simulink model "Test_RC_Filters"  (R2017b)
settings: Solver=VariableStepAuto  StartTime=0.0  StopTime=1  MaxStep=1e-4  RelTol=1e-3
libraries: powerlib x48, powerlib_extras x2
settings Model: Creator=chemi  LastModifiedBy=chemi

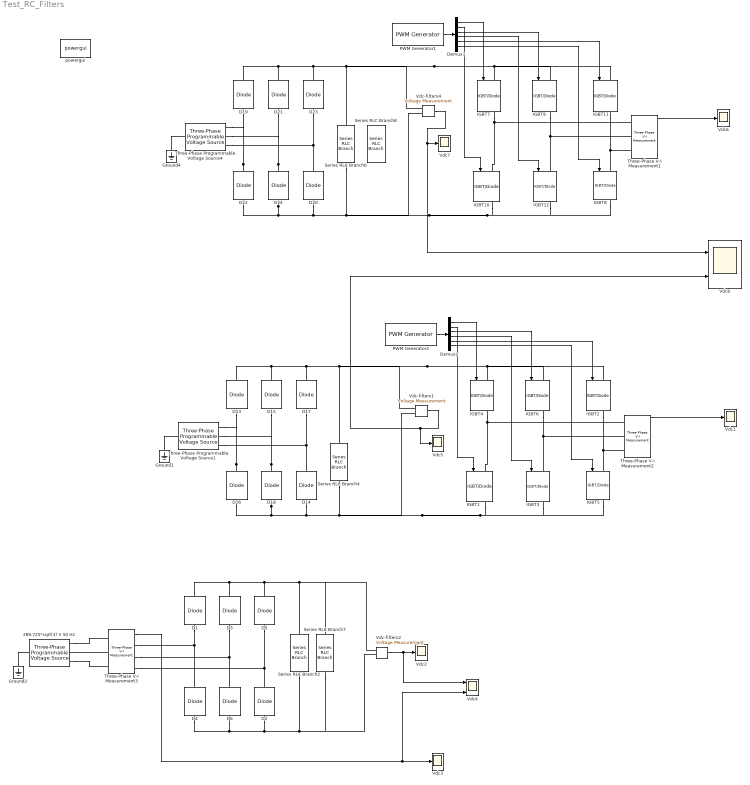
== system Test_RC_Filters ==
  289.725*sqrt(3) V 50 Hz : powerlib/Electrical Sources/Three-Phase Programmable Voltage Source  PositiveSequence=[289.725*sqrt(3) 0 50]  VariationEntity=None  VariationType=Table of time-amplitude pairs  VariationTypeAlt=Step  VariationStep=0.5  VariationRate=10  VariationMagnitude=0.3  VariationFrequency=2  VariationTiming=[1 2]  VariationPhaseA=off  Amplitudes=[1 0.8 1.2 1.0]  TimeValues=[0 0.1 0.15 0.2]  HarmonicGeneration=off  HarmonicA=[3 0.2 -25 0]  HarmonicB=[2 0.15 35 2]  Timing="[0.05  3]"  BusType=swing  Pref=0  Qref=0  Qmin=-inf  Qmax=inf
  D{1..6,13..24} (18 alike) : powerlib/Power Electronics/Diode  Ron=0.001  Lon=0  Vf=0  IC=0  UseSnubber=off  Rs=500  Cs=250e-9  Measurements=off
  Demux1 : Demux  Outputs=6
  Demux2 : Demux  Outputs=6
  Ground1 : powerlib/Elements/Ground  LConnTagsString=a
  Ground2 : powerlib/Elements/Ground  LConnTagsString=a
  Ground4 : powerlib/Elements/Ground  LConnTagsString=a
  IGBT{1..12} (12 alike) : powerlib/Power Electronics/IGBT//Diode  Ron=1e-3  Rs=1e5  Cs=inf  Measurements=on
  PWM Generator1 : powerlib_extras/Control  Blocks/PWM Generator  GeneratorMode="3-arm  bridge (6 pulses)"  Fc=5000  Internal=on  mIndex=1  Freq=50  Phase=0
  PWM Generator2 : powerlib_extras/Control  Blocks/PWM Generator  GeneratorMode="3-arm  bridge (6 pulses)"  Fc=5000  Internal=on  mIndex=1  Freq=50  Phase=0
  Series RLC Branch2 : powerlib/Elements/Series RLC Branch  LConnTagsString=__new0  RConnTagsString=__new0  BranchType=C  Resistance=3000  Inductance=200e-6  SetiL0=off  InitialCurrent=0  Capacitance=22000e-6  Setx0=off  InitialVoltage=0  Measurements=None
  Series RLC Branch4 : powerlib/Elements/Series RLC Branch  LConnTagsString=__new0  RConnTagsString=__new0  BranchType=C  Resistance=3000  Inductance=1e-3  SetiL0=off  InitialCurrent=0  Capacitance=3500e-6  Setx0=off  InitialVoltage=0  Measurements=None
  Series RLC Branch6 : powerlib/Elements/Series RLC Branch  LConnTagsString=__new0  RConnTagsString=__new0  BranchType=C  Resistance=3000  Inductance=1e-3  SetiL0=off  InitialCurrent=0  Capacitance=17000e-6  Setx0=off  InitialVoltage=0  Measurements=None
  Series RLC Branch7 : powerlib/Elements/Series RLC Branch  LConnTagsString=__new0  RConnTagsString=__new0  BranchType=R  Resistance=2200  Inductance=200e-6  SetiL0=off  InitialCurrent=0  Capacitance=10000e-6  Setx0=off  InitialVoltage=0  Measurements=None
  Series RLC Branch8 : powerlib/Elements/Series RLC Branch  LConnTagsString=__new0  RConnTagsString=__new0  BranchType=R  Resistance=3000  Inductance=200e-6  SetiL0=off  InitialCurrent=0  Capacitance=10000e-6  Setx0=off  InitialVoltage=0  Measurements=None
  Three-Phase Programmable Voltage Source1 : powerlib/Electrical Sources/Three-Phase Programmable Voltage Source  PositiveSequence=[289.725*sqrt(3) 0 50]  VariationEntity=None  VariationType=Table of time-amplitude pairs  VariationTypeAlt=Step  VariationStep=0.5  VariationRate=10  VariationMagnitude=0.3  VariationFrequency=2  VariationTiming=[1 2]  VariationPhaseA=off  Amplitudes=[1 0.8 1.2 1.0]  TimeValues=[0 0.1 0.15 0.2]  HarmonicGeneration=off  HarmonicA=[3 0.2 -25 0]  HarmonicB=[2 0.15 35 2]  Timing="[0.05  3]"  BusType=swing  Pref=0  Qref=0  Qmin=-inf  Qmax=inf
  Three-Phase Programmable Voltage Source4 : powerlib/Electrical Sources/Three-Phase Programmable Voltage Source  PositiveSequence=[289.725*sqrt(3) 0 50]  VariationEntity=None  VariationType=Table of time-amplitude pairs  VariationTypeAlt=Step  VariationStep=0.5  VariationRate=10  VariationMagnitude=0.3  VariationFrequency=2  VariationTiming=[1 2]  VariationPhaseA=off  Amplitudes=[1 0.8 1.2 1.0]  TimeValues=[0 0.1 0.15 0.2]  HarmonicGeneration=off  HarmonicA=[3 0.2 -25 0]  HarmonicB=[2 0.15 35 2]  Timing="[0.05  3]"  BusType=swing  Pref=0  Qref=0  Qmin=-inf  Qmax=inf
  Three-Phase V-I Measurement1 : powerlib/Measurements/Three-Phase V-I Measurement  VoltageMeasurement=phase-to-phase  SetLabelV=off  LabelV=Vabc  Vpu=off  VpuLL=off  CurrentMeasurement=yes  SetLabelI=off  LabelI=Iabc  Ipu=off  Pbase=100e6  Vbase=500e3  OutputType=Complex  PhasorSimulation=off  PSBequivalent=0
  Three-Phase V-I Measurement2 : powerlib/Measurements/Three-Phase V-I Measurement  VoltageMeasurement=phase-to-phase  SetLabelV=off  LabelV=Vabc  Vpu=off  VpuLL=off  CurrentMeasurement=yes  SetLabelI=off  LabelI=Iabc  Ipu=off  Pbase=100e6  Vbase=500e3  OutputType=Complex  PhasorSimulation=off  PSBequivalent=0
  Three-Phase V-I Measurement3 : powerlib/Measurements/Three-Phase V-I Measurement  VoltageMeasurement=phase-to-phase  SetLabelV=off  LabelV=Vabc  Vpu=off  VpuLL=off  CurrentMeasurement=no  SetLabelI=off  LabelI=Iabc  Ipu=off  Pbase=100e6  Vbase=500e3  OutputType=Complex  PhasorSimulation=off  PSBequivalent=0
  Vdc-filters1 : powerlib/Measurements/Voltage Measurement  PhasorSimulation=off  OutputType=Complex  PSBequivalent=0
  Vdc-filters2 : powerlib/Measurements/Voltage Measurement  PhasorSimulation=off  OutputType=Complex  PSBequivalent=0
  Vdc-filters4 : powerlib/Measurements/Voltage Measurement  PhasorSimulation=off  OutputType=Complex  PSBequivalent=0
  Vdc{1..3,5..7} (6 alike) : Scope
  Vdc4 : Scope  NumInputPorts=2
  Vdc8 : Scope  NumInputPorts=2
  powergui : powerlib/powergui  Priority=1  SimulationMode=Continuous  SampleTime=50e-6  frequency=60  Iterations=50  frequencyindice=50  Pbase=100e6  ErrMax=1e-4  UnitsV=kV  UnitsW=MW  buscounter=0  FunctionMessages=off  echomessages=off  EnableUseOfTLC=off  CurrentSourceSwitches=off  DisableSnubberDevices=off  DisableRonSwitches=off  DisableVfSwitches=off  DisplayEquations=off  SolverType=Tustin/Backward Euler (TBE)  Interpol=off  ExternalGateDelay=off  methode=off  Ts=100  x0status=blocks  SPID=on  SwTol=0  HookPort=off  RestoreLinks=warning  ResistiveCurrentMeasurement=off  Frange=[0:2:500]  Ylog=off  Xlog=on  ShowGrid=off  save=off  variable=ZData  structure=0  ZoomFFT=on  StartTime=0.0  cycles=1  DisplayStyle=1  fundamental=60  FreqAxis=off  MaxFrequency=1000  frequencyindicesteady=1  RmsSteady=1  display=off
  wires:
  Vdc-filters4/1 -> Vdc7/1, Vdc8/1
  Three-Phase V-I Measurement1/1 -> Vdc6/1
  Demux1/5 -> IGBT11/1
  Demux1/2 -> IGBT10/1
  Demux1/4 -> IGBT12/1
  Demux1/1 -> IGBT7/1
  Demux1/3 -> IGBT9/1
  PWM Generator1/1 -> Demux1/1
  Demux1/6 -> IGBT8/1
  Demux2/6 -> IGBT5/1
  PWM Generator2/1 -> Demux2/1
  Demux2/3 -> IGBT6/1
  Demux2/1 -> IGBT4/1
  Demux2/4 -> IGBT3/1
  Demux2/2 -> IGBT1/1
  Demux2/5 -> IGBT2/1
  Three-Phase V-I Measurement2/1 -> Vdc1/1
  Vdc-filters1/1 -> Vdc8/2, Vdc5/1
  Vdc-filters2/1 -> Vdc4/1, Vdc2/1
  Three-Phase V-I Measurement3/1 -> Vdc4/2, Vdc3/1
  connections:
  D23/RConn1 -- Vdc-filters4/LConn1 -- IGBT7/LConn1 -- IGBT11/LConn1 -- IGBT9/LConn1 -- Series RLC Branch6/LConn1 -- D21/RConn1 -- D19/RConn1
  D24/LConn1 -- D20/LConn1 -- IGBT8/RConn1 -- IGBT12/RConn1 -- IGBT10/RConn1 -- Vdc-filters4/LConn2 -- Series RLC Branch6/RConn1 -- D22/LConn1
  Three-Phase V-I Measurement1/LConn1 -- IGBT10/LConn1 -- IGBT7/RConn1
  Three-Phase V-I Measurement1/LConn2 -- IGBT12/LConn1 -- IGBT9/RConn1
  Three-Phase V-I Measurement1/LConn3 -- IGBT8/LConn1 -- IGBT11/RConn1
  D23/LConn1 -- D20/RConn1 -- Three-Phase Programmable Voltage Source4/RConn3
  D24/RConn1 -- D21/LConn1 -- Three-Phase Programmable Voltage Source4/RConn2
  D22/RConn1 -- D19/LConn1 -- Three-Phase Programmable Voltage Source4/RConn1
  Ground4/LConn1 -- Three-Phase Programmable Voltage Source4/LConn1
  D17/RConn1 -- D13/RConn1 -- D15/RConn1 -- IGBT6/LConn1 -- IGBT2/LConn1 -- IGBT4/LConn1 -- Vdc-filters1/LConn1 -- Series RLC Branch4/LConn1
  D18/LConn1 -- D16/LConn1 -- Vdc-filters1/LConn2 -- IGBT1/RConn1 -- IGBT3/RConn1 -- IGBT5/RConn1 -- Series RLC Branch4/RConn1 -- D14/LConn1
  Three-Phase V-I Measurement2/LConn1 -- IGBT4/RConn1 -- IGBT1/LConn1
  Three-Phase V-I Measurement2/LConn2 -- IGBT6/RConn1 -- IGBT3/LConn1
  Three-Phase V-I Measurement2/LConn3 -- IGBT2/RConn1 -- IGBT5/LConn1
  D17/LConn1 -- Three-Phase Programmable Voltage Source1/RConn3 -- D14/RConn1
  D18/RConn1 -- Three-Phase Programmable Voltage Source1/RConn2 -- D15/LConn1
  D16/RConn1 -- Three-Phase Programmable Voltage Source1/RConn1 -- D13/LConn1
  Ground1/LConn1 -- Three-Phase Programmable Voltage Source1/LConn1
  D5/RConn1 -- Series RLC Branch2/LConn1 -- Series RLC Branch7/LConn1 -- Vdc-filters2/LConn1 -- D1/RConn1 -- D3/RConn1
  D3/LConn1 -- Three-Phase V-I Measurement3/RConn2 -- D6/RConn1
  Series RLC Branch2/RConn1 -- Vdc-filters2/LConn2 -- Series RLC Branch7/RConn1 -- D2/LConn1 -- D4/LConn1 -- D6/LConn1
  D1/LConn1 -- Three-Phase V-I Measurement3/RConn1 -- D4/RConn1
  D5/LConn1 -- Three-Phase V-I Measurement3/RConn3 -- D2/RConn1
  Ground2/LConn1 -- 289.725*sqrt(3) V 50 Hz/LConn1
  Three-Phase V-I Measurement3/LConn2 -- 289.725*sqrt(3) V 50 Hz/RConn2
  289.725*sqrt(3) V 50 Hz/RConn1 -- Three-Phase V-I Measurement3/LConn1
  289.725*sqrt(3) V 50 Hz/RConn3 -- Three-Phase V-I Measurement3/LConn3
